simulink model "IM_neuron"  (Simulink 8.3)
settings: Solver=ode45  StartTime=0.0  StopTime=200  RelTol=1e-3
values from neighbouring files (symbols this model uses):
  a = 0.02    [test_IM_neuron.m]
  b = 0.2    [test_IM_neuron.m]
  c = -50    [test_IM_neuron.m]
  c1 = 0.04    [test_IM_neuron.m]
  c2 = 5    [test_IM_neuron.m]
  c3 = 140    [test_IM_neuron.m]
  c4 = 1    [test_IM_neuron.m]
  c5 = 1    [test_IM_neuron.m]
  d = 2    [test_IM_neuron.m]
  syn_i = 10    [test_IM_neuron.m]
  vth = 30    [test_IM_neuron.m]    (also in test_hp_memristor.m = 0; test_memristor.m = 0)
libraries: simulink x1
settings Model: Creator=wjj  LastModifiedBy=wjj  SimulationMode=accelerator
settings DataIOCC: SignalLoggingSaveFormat=Dataset
settings DebuggingCC: UnderspecifiedInitializationDetection=Simplified  StateNameClashWarn=none
settings GRTTargetCC: CombineOutputUpdateFcns=on  GRTInterface=off

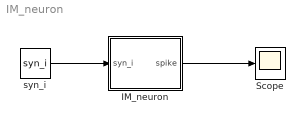
== system IM_neuron ==
  IM_neuron : Subsystem
  Scope : Scope
  syn_i : Constant  Value=syn_i
  wires:
  syn_i/1 -> IM_neuron/1(syn_i)
  IM_neuron/1(spike) -> Scope/1

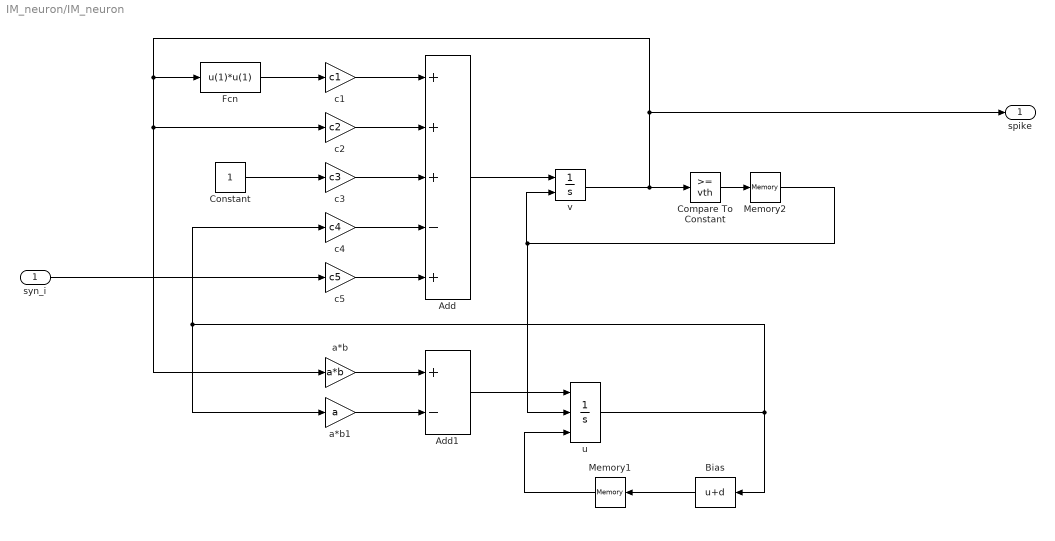
== system IM_neuron/IM_neuron ==
  syn_i : Inport
  Add : Sum  Inputs=+++-+
  Add1 : Sum  Inputs=+-
  Bias : Bias  Bias=d
  Compare To Constant : simulink/Logic and Bit Operations/Compare To Constant  relop=>=  const=vth  OutDataTypeStr=boolean
  Constant : Constant
  Fcn : Fcn  Expr=u(1)*u(1)
  Memory1 : Memory
  Memory2 : Memory
  a*b : Gain  Gain=a*b
  a*b1 : Gain  Gain=a
  c1 : Gain  Gain=c1
  c2 : Gain  Gain=c2
  c3 : Gain  Gain=c3
  c4 : Gain  Gain=c4
  c5 : Gain  Gain=c5
  u : Integrator  ExternalReset=rising  InitialConditionSource=external
  v : Integrator  ExternalReset=rising  InitialCondition=c
  spike : Outport
  wires:
  Bias/1 -> Memory1/1
  a*b1/1 -> Add1/2
  Memory1/1 -> u/3
  Fcn/1 -> c1/1
  Add/1 -> v/1
  c5/1 -> Add/5
  v/1 -> spike/1, a*b/1, c2/1, Fcn/1, Compare To Constant/1
  u/1 -> a*b1/1, c4/1, Bias/1
  c4/1 -> Add/4
  c3/1 -> Add/3
  a*b/1 -> Add1/1
  Add1/1 -> u/1
  syn_i/1 -> c5/1
  c1/1 -> Add/1
  c2/1 -> Add/2
  Constant/1 -> c3/1
  Memory2/1 -> u/2, v/2
  Compare To Constant/1 -> Memory2/1
